simulink subsystem "motor"  (R2023a)
settings: Solver=VariableStepAuto  StartTime=0.0  StopTime=10.0  RelTol=1e-3
settings Model: Creator=lehas  LastModifiedBy=lehas

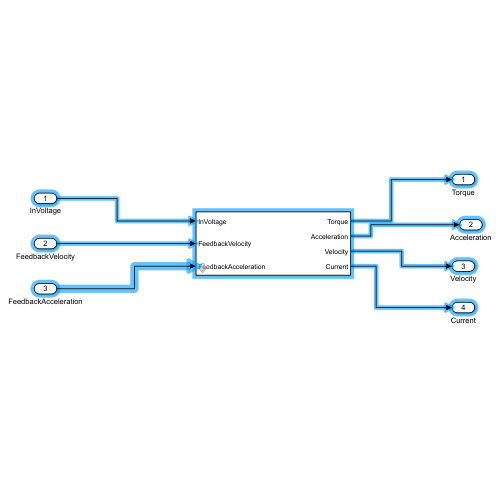
[thumbnail: Simulink's stored preview of the top-level diagram]
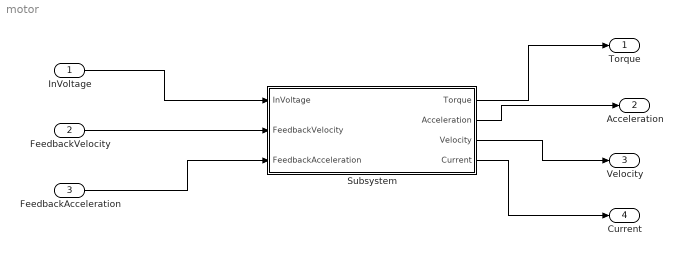
== system motor ==
  InVoltage : Inport
  FeedbackVelocity : Inport  Port=2
  FeedbackAcceleration : Inport  Port=3
  Subsystem : Subsystem  mask{L=3.5e-04, R=10, km=0.016, kw=62.83, J_motor=5e-07, vis_friction_coef_motor=2.4e-05}
      mask prompts: L "Rotor inductance, H"; R "Rotor resistance, Ohm"; km "Torque constant"; kw "Speed constant"; J_motor "Motor inertia, kg * m^2"; vis_friction_coef_motor "viscous friction coefficient, kg * m^2 / s"
  Torque : Outport
  Acceleration : Outport  Port=2
  Velocity : Outport  Port=3
  Current : Outport  Port=4
  wires:
  Subsystem/4(Current) -> Current/1
  Subsystem/2(Acceleration) -> Acceleration/1
  Subsystem/1(Torque) -> Torque/1
  InVoltage/1 -> Subsystem/1(InVoltage)
  Subsystem/3(Velocity) -> Velocity/1
  FeedbackVelocity/1 -> Subsystem/2(FeedbackVelocity)
  FeedbackAcceleration/1 -> Subsystem/3(FeedbackAcceleration)

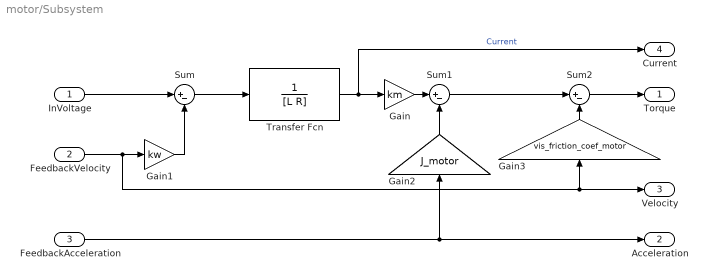
== system motor/Subsystem ==
  InVoltage : Inport
  FeedbackVelocity : Inport  Port=2
  FeedbackAcceleration : Inport  Port=3
  Gain : Gain  Gain=km
  Gain1 : Gain  Gain=kw
  Gain2 : Gain  Gain=J_motor
  Gain3 : Gain  Gain=vis_friction_coef_motor
  Sum : Sum  Inputs=|+-
  Sum1 : Sum  Inputs=|+-
  Sum2 : Sum  Inputs=|+-
  Transfer Fcn : TransferFcn  Denominator=[L R]
  Torque : Outport
  Acceleration : Outport  Port=2
  Velocity : Outport  Port=3
  Current : Outport  Port=4
  wires:
  Transfer Fcn/1 -> Current/1, Gain/1  "Current"
  Gain/1 -> Sum1/1
  InVoltage/1 -> Sum/1
  Sum2/1 -> Torque/1
  Sum/1 -> Transfer Fcn/1
  FeedbackVelocity/1 -> Velocity/1, Gain3/1, Gain1/1
  Gain3/1 -> Sum2/2
  FeedbackAcceleration/1 -> Acceleration/1, Gain2/1
  Gain1/1 -> Sum/2
  Sum1/1 -> Sum2/1
  Gain2/1 -> Sum1/2
